simulink model "LAB2_BOILER_MODEL"  (R2018a)
settings: Solver=VariableStepAuto  StartTime=0.0  StopTime=10.0  RelTol=1e-3
undefined symbols (not defined in the file): fv1, fv2, j1, J1, j2, J2, K1, K2, mwo_setpoint, MWOFR, MWOTV, N1, N2, tp_setpoint, TPFR, TPTV
settings Model: Creator=zchen61  LastModifiedBy=zchen61
settings CodeAppCC: StateflowObjectComments=on

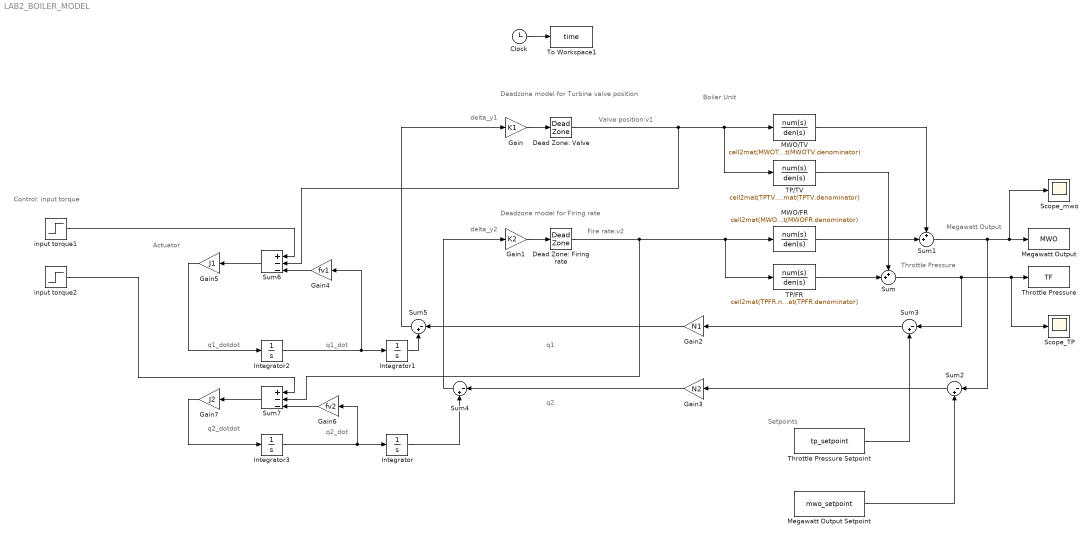
== system LAB2_BOILER_MODEL ==
  note: Control: input torque
  note: Actuator
  note: Boiler Unit
  note: Setpoints
  note: Deadzone model for Firing rate
  note: Deadzone model for Turbine valve position
  note: delta_y1
  note: Throttle Pressure
  note: Megawatt Output
  note: Valve position:v1
  note: Fire rate:v2
  note: delta_y2
  note: q1
  note: q2
  note: q1_dot
  note: q2_dot
  note: q1_dotdot
  note: q2_dotdot
  Clock : Clock
  Dead Zone: Firing rate : DeadZone  LowerValue=-K2*j2  UpperValue=K2*j2  SaturateOnIntegerOverflow=on
  Dead Zone: Valve : DeadZone  LowerValue=-K1*j1  UpperValue=K1*j1  SaturateOnIntegerOverflow=on
  Gain : Gain  Gain=K1
  Gain1 : Gain  Gain=K2
  Gain2 : Gain  Gain=N1
  Gain3 : Gain  Gain=N2
  Gain4 : Gain  Gain=fv1
  Gain5 : Gain  Gain=J1
  Gain6 : Gain  Gain=fv2
  Gain7 : Gain  Gain=J2
  Integrator{,1..3} (4 alike) : Integrator
  MWO/FR : TransferFcn  Numerator=cell2mat(MWOFR.numerator)  Denominator=cell2mat(MWOFR.denominator)
  MWO/TV : TransferFcn  Numerator=cell2mat(MWOTV.numerator)  Denominator=cell2mat(MWOTV.denominator)
  "Megawatt Output " : ToWorkspace  VariableName=MWO  SampleTime=-1
  Megawatt Output Setpoint : Constant  Value=mwo_setpoint
  Scope_TP : Scope
  Scope_mwo : Scope
  Sum : Sum  Inputs=++|
  Sum1 : Sum  Inputs=++|
  Sum{2..5} (4 alike) : Sum  Inputs=|-+
  Sum6 : Sum  Inputs=|+|-|-
  Sum7 : Sum  Inputs=|+|-|-
  TP/FR : TransferFcn  Numerator=cell2mat(TPFR.numerator)  Denominator=cell2mat(TPFR.denominator)
  TP/TV : TransferFcn  Numerator=cell2mat(TPTV.numerator)  Denominator=cell2mat(TPTV.denominator)
  Throttle Pressure : ToWorkspace  VariableName=TF  SampleTime=-1
  "Throttle Pressure Setpoint " : Constant  Value=tp_setpoint
  To Workspace1 : ToWorkspace  VariableName=time  SampleTime=-1
  input torque1 : Step  SampleTime=0
  input torque2 : Step  SampleTime=0
  wires:
  MWO/TV/1 -> Sum1/1
  Dead Zone: Firing rate/1 -> TP/FR/1, MWO/FR/1, Sum7/2
  TP/FR/1 -> Sum/2
  TP/TV/1 -> Sum/1
  MWO/FR/1 -> Sum1/2
  Dead Zone: Valve/1 -> Sum6/2, MWO/TV/1, TP/TV/1
  Sum/1 -> Sum3/1, Scope_TP/1, Throttle Pressure/1
  Sum1/1 -> Sum2/1, Scope_mwo/1, "Megawatt Output "/1
  Sum5/1 -> Gain/1
  Gain/1 -> Dead Zone: Valve/1
  Clock/1 -> To Workspace1/1
  Sum4/1 -> Gain1/1
  Gain1/1 -> Dead Zone: Firing rate/1
  Megawatt Output Setpoint/1 -> Sum2/2
  "Throttle Pressure Setpoint "/1 -> Sum3/2
  Sum2/1 -> Gain3/1
  Sum3/1 -> Gain2/1
  Integrator1/1 -> Sum5/2
  Integrator/1 -> Sum4/2
  Gain3/1 -> Sum4/1
  Gain2/1 -> Sum5/1
  Integrator2/1 -> Gain4/1, Integrator1/1
  Integrator3/1 -> Gain6/1, Integrator/1
  Gain4/1 -> Sum6/3
  input torque1/1 -> Sum6/1
  Sum6/1 -> Gain5/1
  Gain5/1 -> Integrator2/1
  Gain6/1 -> Sum7/3
  Sum7/1 -> Gain7/1
  Gain7/1 -> Integrator3/1
  input torque2/1 -> Sum7/1
